simulink model "vrmaglev"  (R2018b)
settings: Solver=ode5  StartTime=0.0  StopTime=5  FixedStep=1e-3  MaxStep=0.001  RelTol=1e-3  AbsTol=1e-5
model workspace (MATLAB code in the model file):
  | Ts=1e-3;
values from neighbouring files (symbols this model uses):
  A = (2 - 3.7887*T) * (2 + 3.9791*T) / 2 / (2 + 10.2083*T)    (= 0.429666937991)    [P3.m]    (also in Transfer.m = [0, 1, 0; 15.0757, -0.1904, 13.1260; 0, 0, -250])
  C1 = (-2-3.7887*T) / (2-3.7887*T)    (= -2.2199378552)    [P3.m]
  C2 = (-2 + 3.9791*T) / (2 + 3.9791*T)    (= -0.430707270139)    [P3.m]
  C3 = (-2 + 10.2083*T) / (2 + 10.2083*T)    (= 0.0103076458683)    [P3.m]
  K_M = 19.0620 * (-1 - p(1)) * (-1 - p(2)) / (-1 - z(1)) / (-1 - z(2))    [P3.m]
  m = 100 + a    (= 105)    [const.m]
  T = 0.2    [P3.m]
  yd = 0.3 + a/100    (= 0.35)    [const.m]
libraries: vrlib x2, simulink x1
Description:
  | Magnetic Levitation Model
  | 
  | vrmaglev is an example showing the interaction between dynamic models in Simulink(R)
  | and virtual worlds. The Simulink model represents the HUMUSOFT(R) CE152 Magnetic Levitation
  | educational / presentation scale model. (http://www.humusoft.com/link/models)
  | 
  | The plant model is controlled by a PID controller with feed forward to cope with the nonlinearity
  | of the magnetic levitation system.
  | 
  | The position of the ball responds to the changing value of the setpoint. You can observe
  | this change not only in the Scope window, but also in a viewer window displaying
  | the virtual world. Note that the position of the ball represents the real dynamics of the system.
  | If you switch the VRML viewer to the Camera 3 viewpoint, you can observe and control the ball easier.
  | 
  | There are two possible methods of setting the ball position setpoint - using a Signal Generator
  | and visually by clicking at a desired position in the virtual reality scene.
  | 
  | In the virtual scene, a VRML sensor is defined. If you click in the space between the magnetic coil
  | and the bottom plate, VRML sensor is updated and its value is read into Simulink model using the
  | VR Source block.
settings Model: FPTRunName=Active  ExtModeTrigDuration=5000  ExtModeTrigLevel=0.500000  Creator=The MathWorks, Inc.  LastModifiedBy=hadiz
settings SolverCC: AutoScaleAbsTol=off
settings DataIOCC: SaveFormat=Array  SaveOutput=off  SaveTime=off  SignalLoggingName=logsOut
settings OptimizationCC: BlockReduction=off  BooleanDataType=off  OptimizeBlockIOStorage=off  BufferReuse=off  GlobalBufferReuse=off  ExpressionFolding=off  ExpressionDepthLimit=2147483647  LocalBlockOutputs=off  InitFltsAndDblsToZero=on  LifeSpan=inf  OptimizeDataStoreBuffers=off  BusAssignmentInplaceUpdate=off
settings DebuggingCC: UnderspecifiedInitializationDetection=Classic  MergeDetectMultiDrivingBlocksExec=none  CheckExecutionContextPreStartOutputMsg=on  SignalResolutionControl=TryResolveAllWithWarning  MultiTaskDSMMsg=warning  MultiTaskCondExecSysMsg=none  FcnCallInpInsideContextMsg=warning  StateNameClashWarn=warning  SFUnexpectedBacktrackingDiag=warning  SFNoUnconditionalDefaultTransitionDiag=warning  SFExecutionAtInitializationDiag=none
settings HardwareCC: ProdBitPerPointer=32  ProdBitPerSizeT=32  ProdBitPerPtrDiffT=32  ProdLargestAtomicFloat=None  ProdIntDivRoundTo=Undefined  ProdEndianess=Unspecified  ProdWordSize=32  ProdHWDeviceType=32-bit Generic  TargetUnknown=on
settings ModelReferenceCC: UpdateModelReferenceTargets=IfOutOfDate  PropagateSignalLabelsOutOfModel=off
settings SFSimCC: SimUseLocalCustomCode=off
settings RTWCC: RetainRTWFile=on  RTWUseLocalCustomCode=off
settings CodeAppCC: StateflowObjectComments=on
settings GRTTargetCC: TargetFcnLib=ansi_tfl_tmw.mat  TargetLangStandard=C89/C90 (ANSI)  CombineOutputUpdateFcns=off  GRTInterface=on
settings ConfigComp: CovMetricSettings=d  CovSaveCumulativeToWorkspaceVar=on  CovSaveSingleToWorkspaceVar=on  CovExternalEMLEnable=off  CovSFcnEnable=off

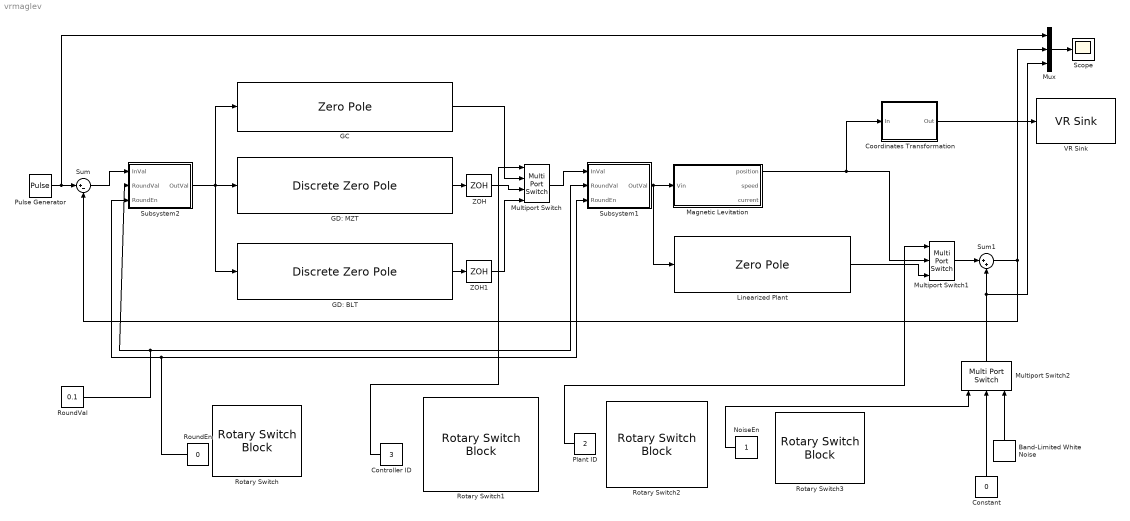
== system vrmaglev ==
  Band-Limited White Noise : simulink/Sources/Band-Limited White Noise  Cov=1e-4 * T  Ts=T  seed=[23341]
  Constant : Constant  Value=0
  Controller ID : Constant  Value=3
  Coordinates Transformation : Subsystem
  GC : ZeroPole  Zeros=[3.7887, -3.9791]  Poles=[0, -10.2083]  Gain=19.0620
  GD: BLT : DiscreteZeroPole  Zeros=[-C1, -C2]  Poles=[1, -C3]  Gain=19.0620 * A  SampleTime=T
  GD: MZT : DiscreteZeroPole  Zeros=[exp(3.7887*T), exp(-3.9791*T)]  Poles=[1, exp(-10.2083*T)]  Gain=K_M  SampleTime=T
  Linearized Plant : ZeroPole  Zeros=[]  Poles=[-250, -3.9791, +3.7887]  Gain=656.3
  Magnetic Levitation : Subsystem
  Multiport Switch : MultiPortSwitch
  Multiport Switch1 : MultiPortSwitch  Inputs=2
  Multiport Switch2 : MultiPortSwitch  DataPortOrder=Zero-based contiguous  Inputs=2  zeroidx=on
  Mux : Mux  Inputs=3
  NoiseEn : Constant
  Plant ID : Constant  Value=2
  Pulse Generator : DiscretePulseGenerator  PulseType=Time based  Amplitude=yd  Period=10  PulseWidth=50
  Rotary Switch : RotarySwitchBlock  WebBlockId=228
      settings: Values={{'Off', 'On'}, [0 1]}
  Rotary Switch1 : RotarySwitchBlock  WebBlockId=212
      settings: Values={{'GC', 'GD: MZT', 'GD: BLT'}, [1 2 3]}
  Rotary Switch2 : RotarySwitchBlock  WebBlockId=211
      settings: Values={{'MagLev', 'Model'}, [1 2]}
  Rotary Switch3 : RotarySwitchBlock  WebBlockId=257
      settings: Values={{'Off', 'On'}, [0 1]}
  RoundEn : Constant  Value=0
  RoundVal : Constant  Value=0.1
  Scope : Scope
  Subsystem1 : Subsystem
  Subsystem2 : Subsystem
  Sum : Sum  Inputs=|+-  SaturateOnIntegerOverflow=on  InputSameDT=on  OutDataTypeStr=Inherit: Same as first input
  Sum1 : Sum  Inputs=|++
  VR Sink : vrlib/VR Sink  InstantiateOnLoad=on  SampleTime=0.02  ViewEnable=on  RemoteChange=off  RemoteView=off  FieldsWritten=Ball.translation.3.1.1.double  WorldFileName=maglev.wrl  WorldDescription=VR Magnetic Levitation Model  AutoView=on  VideoDimensions=[]  AllowVariableSize=off
      settings: SourceProductBaseCode=VR
  ZOH : ZeroOrderHold  SampleTime=T
  ZOH1 : ZeroOrderHold  SampleTime=T
  wires:
  Mux/1 -> Scope/1
  Coordinates Transformation/1(Out) -> VR Sink/1
  Magnetic Levitation/1(position) -> Multiport Switch1/2, Coordinates Transformation/1(In)
  Pulse Generator/1 -> Sum/1, Mux/1
  GC/1 -> Multiport Switch/2
  ZOH/1 -> Multiport Switch/3
  Controller ID/1 -> Multiport Switch/1
  ZOH1/1 -> Multiport Switch/4
  GD: MZT/1 -> ZOH/1
  GD: BLT/1 -> ZOH1/1
  Linearized Plant/1 -> Multiport Switch1/3
  Plant ID/1 -> Multiport Switch1/1
  RoundVal/1 -> Subsystem1/2(RoundVal), Subsystem2/2(RoundVal)
  RoundEn/1 -> Subsystem1/3(RoundEn), Subsystem2/3(RoundEn)
  Multiport Switch/1 -> Subsystem1/1(InVal)
  Subsystem1/1(OutVal) -> Linearized Plant/1, Magnetic Levitation/1(Vin)
  Subsystem2/1(OutVal) -> GD: MZT/1, GD: BLT/1, GC/1
  Sum/1 -> Subsystem2/1(InVal)
  Multiport Switch1/1 -> Sum1/1
  Sum1/1 -> Mux/2, Sum/2
  Constant/1 -> Multiport Switch2/2
  Band-Limited White Noise/1 -> Multiport Switch2/3
  Multiport Switch2/1 -> Mux/3, Sum1/2
  NoiseEn/1 -> Multiport Switch2/1

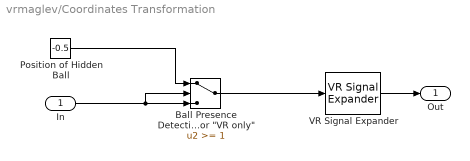
== system vrmaglev/Coordinates Transformation ==
  In : Inport
  "Ball Presence Detection Value > Threshold = Ball Not Present 1 for \"VR only\"" : Switch  Threshold=1  InputSameDT=on
  Position of Hidden Ball : Constant  Value=-0.5
  VR Signal Expander : vrlib/VR Signal Expander  outwidth=3  outidx=[2]
      settings: SourceProductName=Simulink 3D Animation  SourceProductBaseCode=VR
  Out : Outport
  wires:
  Position of Hidden Ball/1 -> "Ball Presence Detection Value > Threshold = Ball Not Present 1 for \"VR only\""/1
  In/1 -> "Ball Presence Detection Value > Threshold = Ball Not Present 1 for \"VR only\""/3, "Ball Presence Detection Value > Threshold = Ball Not Present 1 for \"VR only\""/2
  "Ball Presence Detection Value > Threshold = Ball Not Present 1 for \"VR only\""/1 -> VR Signal Expander/1
  VR Signal Expander/1 -> Out/1

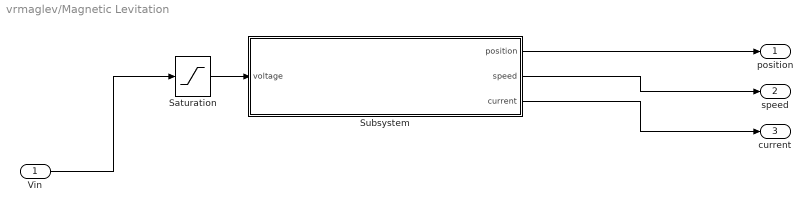
== system vrmaglev/Magnetic Levitation ==
  Vin : Inport
  Saturation : Saturate  UpperLimit=10  LowerLimit=0  ZeroCross=off
  Subsystem : Subsystem
  position : Outport
  speed : Outport  Port=2
  current : Outport  Port=3
  wires:
  Vin/1 -> Saturation/1
  Saturation/1 -> Subsystem/1(voltage)
  Subsystem/1("position ") -> position/1
  Subsystem/2(speed) -> speed/1
  Subsystem/3(current) -> current/1

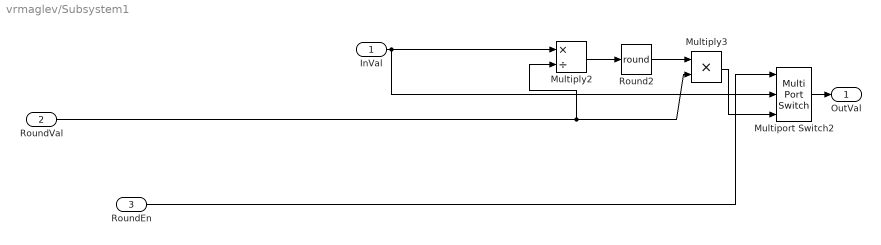
== system vrmaglev/Subsystem1 ==
  InVal : Inport
  RoundVal : Inport  Port=2
  RoundEn : Inport  Port=3
  Multiply2 : Product  Inputs=*/
  Multiply3 : Product  Inputs=**
  Multiport Switch2 : MultiPortSwitch  DataPortOrder=Zero-based contiguous  Inputs=2  zeroidx=on
  Round2 : Rounding  Operator=round
  OutVal : Outport
  wires:
  Multiport Switch2/1 -> OutVal/1
  Round2/1 -> Multiply3/1
  RoundVal/1 -> Multiply3/2, Multiply2/2
  RoundEn/1 -> Multiport Switch2/1
  Multiply2/1 -> Round2/1
  Multiply3/1 -> Multiport Switch2/3
  InVal/1 -> Multiport Switch2/2, Multiply2/1

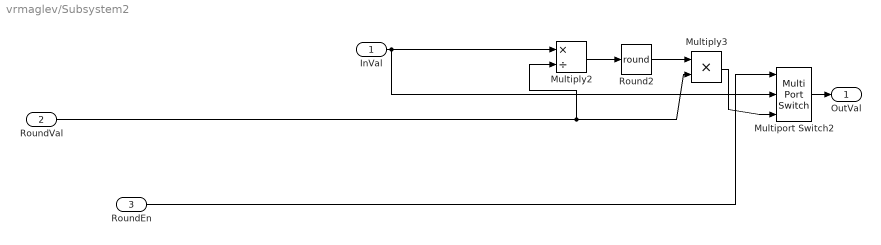
== system vrmaglev/Subsystem2 ==
  InVal : Inport
  RoundVal : Inport  Port=2
  RoundEn : Inport  Port=3
  Multiply2 : Product  Inputs=*/
  Multiply3 : Product  Inputs=**
  Multiport Switch2 : MultiPortSwitch  DataPortOrder=Zero-based contiguous  Inputs=2  zeroidx=on
  Round2 : Rounding  Operator=round
  OutVal : Outport
  wires:
  Multiport Switch2/1 -> OutVal/1
  Round2/1 -> Multiply3/1
  RoundVal/1 -> Multiply3/2, Multiply2/2
  RoundEn/1 -> Multiport Switch2/1
  Multiply2/1 -> Round2/1
  Multiply3/1 -> Multiport Switch2/3
  InVal/1 -> Multiport Switch2/2, Multiply2/1

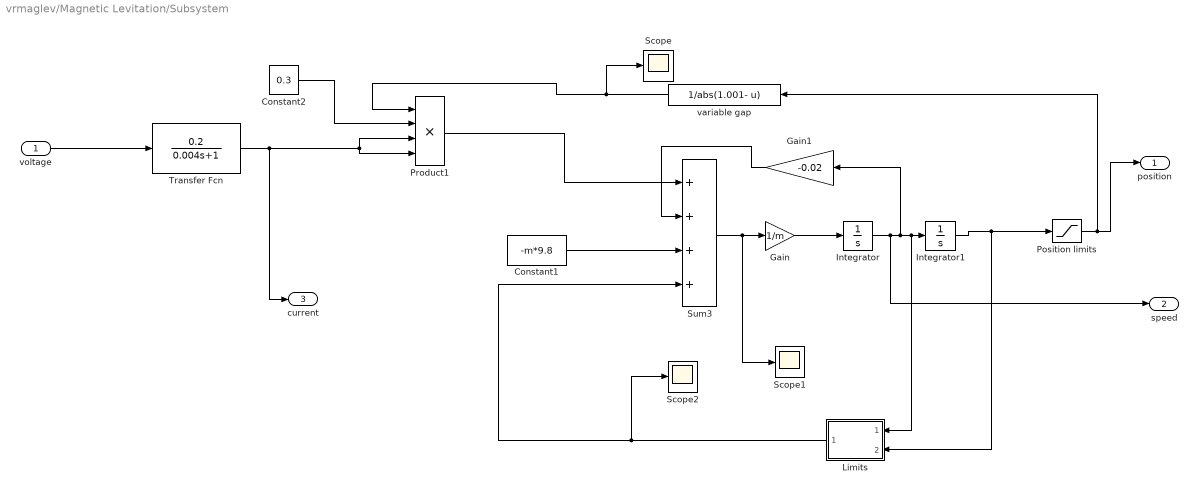
== system vrmaglev/Magnetic Levitation/Subsystem ==
  voltage : Inport
  Constant1 : Constant  Value=-m*9.8
  Constant2 : Constant  Value=0.3
  Gain : Gain  Gain=1/m
  Gain1 : Gain  Gain=-0.02
  Integrator : Integrator
  Integrator1 : Integrator  LimitOutput=on  UpperSaturationLimit=1  LowerSaturationLimit=0
  Limits : Subsystem
      mask Display: disp('LIMIT')
  Position limits : Saturate  UpperLimit=0.998  LowerLimit=0.001  ZeroCross=off
  Product1 : Product  Inputs=4
  Scope : Scope
  Scope1 : Scope
  Scope2 : Scope
  Sum3 : Sum  Inputs=++++
  Transfer Fcn : TransferFcn  Numerator=[0.2]  Denominator=[0.004 1]
  variable gap : Fcn  Expr=1/abs(1.001- u)
  "position " : Outport
  speed : Outport  Port=2
  current : Outport  Port=3
  wires:
  Position limits/1 -> variable gap/1, "position "/1
  Integrator1/1 -> Limits/2(position), Position limits/1
  Sum3/1 -> Scope1/1, Gain/1
  Constant2/1 -> Product1/2
  Constant1/1 -> Sum3/3
  variable gap/1 -> Scope/1, Product1/1
  Gain1/1 -> Sum3/2
  Gain/1 -> Integrator/1
  Integrator/1 -> speed/1, Limits/1(velocity), Integrator1/1, Gain1/1
  Product1/1 -> Sum3/1
  Transfer Fcn/1 -> current/1, Product1/3, Product1/4
  voltage/1 -> Transfer Fcn/1
  Limits/1(force) -> Scope2/1, Sum3/4

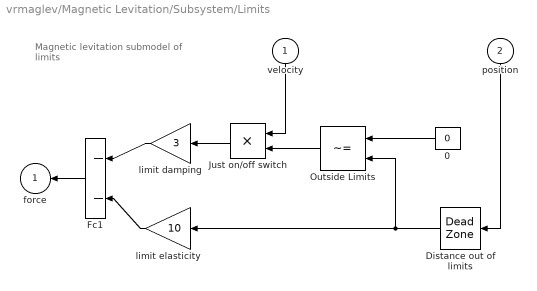
== system vrmaglev/Magnetic Levitation/Subsystem/Limits ==
  note: Magnetic levitation
      | submodel of limits
  velocity : Inport
  position : Inport  Port=2
  0 : Constant  Value=0
  Distance out of limits : DeadZone  LowerValue=0.002  UpperValue=1  ZeroCross=off  SaturateOnIntegerOverflow=on
  Fc1 : Sum  Inputs=--  SaturateOnIntegerOverflow=on  InputSameDT=on  OutDataTypeStr=Inherit: Same as first input
  "Just on/off switch " : Product  SaturateOnIntegerOverflow=on  InputSameDT=on  OutDataTypeStr=Inherit: Same as first input
  Outside Limits : RelationalOperator  Operator=~=  RndMeth=Nearest  InputSameDT=on
  limit damping : Gain  Gain=3  SaturateOnIntegerOverflow=on  OutDataTypeStr=Inherit: Same as input  ParamDataTypeStr=Inherit: Same as input
  limit elasticity : Gain  Gain=10  SaturateOnIntegerOverflow=on  OutDataTypeStr=Inherit: Same as input  ParamDataTypeStr=Inherit: Same as input
  force : Outport
  wires:
  Distance out of limits/1 -> Outside Limits/2, limit elasticity/1
  limit damping/1 -> Fc1/1
  limit elasticity/1 -> Fc1/2
  Outside Limits/1 -> "Just on/off switch "/2
  0/1 -> Outside Limits/1
  "Just on/off switch "/1 -> limit damping/1
  velocity/1 -> "Just on/off switch "/1
  Fc1/1 -> force/1
  position/1 -> Distance out of limits/1
